simulink model "q_3d_crane_cal"  (Simulink 6.6)
settings: Solver=FixedStepDiscrete  StartTime=0.0  StopTime=inf  FixedStep=0.001  RelTol=1e-3
values from neighbouring files (symbols this model uses):
  calib_theta = 4.5*pi/180    (= 0.0785398163397)    [setup_3d_crane.m]
  calib_theta_dot = 1/1000    (= 0.001)    [setup_3d_crane.m]
  calib_x = 2/100    (= 0.02)    [setup_3d_crane.m]
  calib_x_dot = 2/1000    (= 0.002)    [setup_3d_crane.m]
  calib_z = 3/100    (= 0.03)    [setup_3d_crane.m]
  calib_z_dot = 5/1000    (= 0.005)    [setup_3d_crane.m]
  IMAX_AMP = 7    [setup_3d_crane.m]
  K_ENC_ALPHA = 2 * pi / (4 * 1024 )    (= 0.00153398078789)    [config_3d_crane.m]
  K_ENC_GAMMA = 2 * pi / (4 * 1024 )    (= 0.00153398078789)    [config_3d_crane.m]
  K_ENC_THETA = 2 * pi / (4 * 1024 ) / Kg_t    (= 1.53398078789e-05)    [config_3d_crane.m]
  K_ENC_X = - Pt / (4 * 1024 ) / Kg_j    [config_3d_crane.m]
  K_ENC_Z = - 2 * pi * r_y_reel / (4 * 1024 ) / Kg_y    [config_3d_crane.m]
  K_J = lqr(A_J,B_J,Q_J,R_J)    [setup_3d_crane.m]
  K_T = lqr(A_T,B_T,Q_T,R_T)    [setup_3d_crane.m]
  Ka = 0.5    [config_3d_crane.m]
  ki = w0^2*p0*(mp*r_y_reel^2+J_phi)/eff_g_y/Kg_y/eff_m_y/Kt_y/r_y_reel    [d_payload_piv_controller.m]
  kp = w0*(2*zeta*p0*J_phi+w0*mp*r_y_reel^2+w0*J_phi+2*zeta*p0*mp*r_y_reel^2)/eff_g_y/Kg_y/eff_m_y/Kt_y/r_y_reel    [d_payload_piv_controller.m]
  kv = (p0*J_phi+2*zeta*w0*mp*r_y_reel^2+2*zeta*w0*J_phi+p0*mp*r_y_reel^2)/eff_g_y/Kg_y/eff_m_y/Kt_y/r_y_reel    [d_payload_piv_controller.m]
  sp_home_payload = -0.7    [setup_3d_crane.m]
  sp_home_tower = 155    [setup_3d_crane.m]
  sp_home_trolley = 0.25    [setup_3d_crane.m]
  VMAX_DAC = 10    [setup_3d_crane.m]
  wf_gamma = 2 * pi * 2.0    (= 12.5663706144)    [setup_3d_crane.m]
  wf_theta = 2 * pi * 50    (= 314.159265359)    [setup_3d_crane.m]
  wf_x = 2 * pi * 50    (= 314.159265359)    [setup_3d_crane.m]
  wf_z = 2 * pi * 50    (= 314.159265359)    [setup_3d_crane.m]
undefined symbols (not defined in the file or in its folder): DiscIntNeverNeededParam, HIL, qc_get_step_size
libraries: quarc_library x21, simulink x14, simulink_extras x4
settings Model: Creator=MLevis  LastModifiedBy=MLevis  SimulationMode=external  ExtModeTrigDuration=25000
settings SolverCC: PositivePriorityOrder=on
settings RTWCC: SystemTargetFile=quarc_windows.tlc  TemplateMakefile=quarc_default_tmf  Description=QuaRC Win32 Target  ProcessScript=quarc_windows_make_rtw_hook
settings STFCustomTargetCC: TargetFcnLib=ansi_tfl_tmw.mat  TargetPreCompLibLocation=C:\DOCUME~1\ALLUSE~1\APPLIC~1\QUARC\lib\2007a\windows\release  GenFloatMathFcnCalls=ANSI_C  SystemTargetFile=quarc_windows.tlc
settings GRTTargetCC: TargetPreCompLibLocation=C:\DOCUME~1\ALLUSE~1\APPLIC~1\QUARC\lib\2007a\windows\release  MatFileLogging=off  ExtMode=on  ExtModeMexFile=quarc_comm

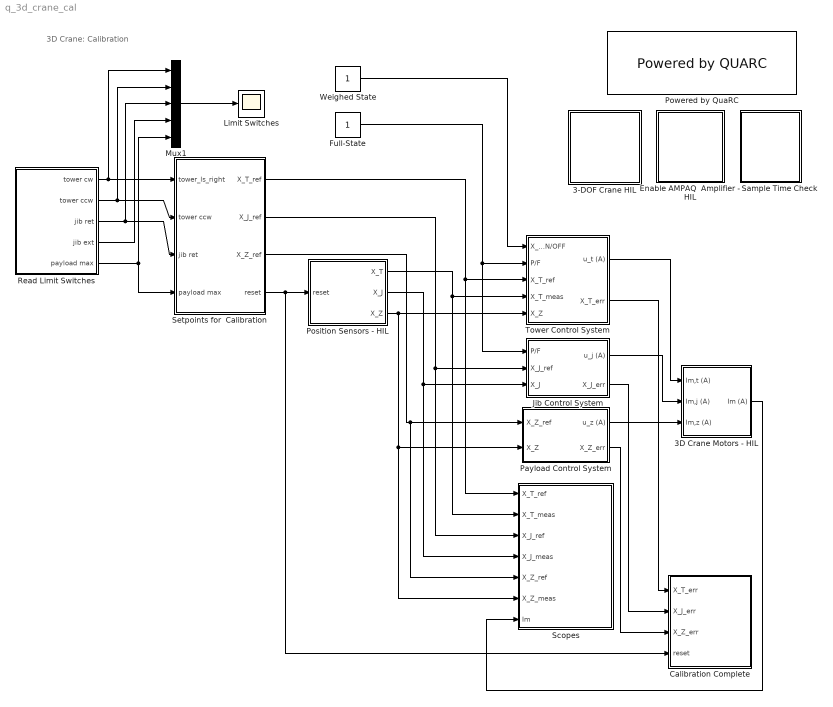
== system q_3d_crane_cal ==
  note: 3D Crane: Calibration
  3-DOF Crane HIL : Subsystem
  3D Crane Motors - HIL : Subsystem
  Calibration Complete : Subsystem
  Enable AMPAQ  Amplifier - HIL : Subsystem
  Full-State : Constant
  Jib Control System : Subsystem
  Limit Switches : Scope
      settings: TimeRange=25  YMin=-1  YMax=2  SaveName=ScopeData4
  Mux1 : Mux  Inputs=5
  Payload Control System : Subsystem
  Position Sensors - HIL : Subsystem
  Powered by QuaRC : quarc_library/Logos/Powered by QUARC  SystemSampleTime=-1
  Read Limit Switches : Subsystem
  Sample Time Check : Subsystem
  Scopes : Subsystem
  Setpoints for  Calibration : Subsystem
  Tower Control System : Subsystem
  Weighed State : Constant
  wires:
  Payload Control System/1(u_z (A)) -> 3D Crane Motors - HIL/3(Im,z (A))
  Tower Control System/1(u_t (A)) -> 3D Crane Motors - HIL/1(Im,t (A))
  Position Sensors - HIL/1(X_T) -> Scopes/2(X_T_meas), Tower Control System/4(X_T_meas)
  Position Sensors - HIL/3(X_Z) -> Scopes/6(X_Z_meas), Payload Control System/2(X_Z), Tower Control System/5(X_Z)
  Position Sensors - HIL/2(X_J) -> Scopes/4(X_J_meas), Jib Control System/3(X_J)
  Setpoints for  Calibration/2(X_J_ref) -> Scopes/3(X_J_ref), Jib Control System/2(X_J_ref)
  Setpoints for  Calibration/1(X_T_ref) -> Scopes/1(X_T_ref), Tower Control System/3(X_T_ref)
  Setpoints for  Calibration/3(X_Z_ref) -> Scopes/5(X_Z_ref), Payload Control System/1(X_Z_ref)
  Jib Control System/1(u_j (A)) -> 3D Crane Motors - HIL/2(Im,j (A))
  Weighed State/1 -> Tower Control System/1(X_W ON/OFF)
  3D Crane Motors - HIL/1(Im (A)) -> Scopes/7(Im)
  Full-State/1 -> Tower Control System/2(P/F), Jib Control System/1(P/F)
  Read Limit Switches/1(tower cw) -> Mux1/1, Setpoints for  Calibration/1(tower_ls_right)
  Read Limit Switches/3(jib ret) -> Mux1/3, Setpoints for  Calibration/3(jib ret)
  Read Limit Switches/5(payload max) -> Setpoints for  Calibration/4(payload max), Mux1/5
  Tower Control System/2(X_T_err) -> Calibration Complete/1(X_T_err)
  Jib Control System/2(X_J_err) -> Calibration Complete/2(X_J_err)
  Payload Control System/2(X_Z_err) -> Calibration Complete/3(X_Z_err)
  Setpoints for  Calibration/4(reset) -> Calibration Complete/4(reset), Position Sensors - HIL/1(reset)
  Read Limit Switches/4(jib ext) -> Mux1/4
  Read Limit Switches/2(tower ccw) -> Mux1/2, Setpoints for  Calibration/2(tower ccw)
  Mux1/1 -> Limit Switches/1

== system q_3d_crane_cal/3-DOF Crane HIL ==
  HIL Initialize : quarc_library/Data Acquisition/Generic/Configuration/HIL Initialize  object_name=HIL-1  board_type=q8  board_number=0  exclusive=off  active=on  hardware_clocks=[]  clock_modes=[]  initial_clock_frequencies=[]  set_clock_params_at_start=on  set_clock_params_at_switch_in=on  set_clock_frequencies_at_start=off  set_clock_frequencies_at_switch_in=off  analog_input_channels=[]  analog_input_maximums=[]  analog_input_minimums=[]  set_analog_input_params_at_start=on  set_analog_input_params_at_switch_in=on  analog_output_channels=[0:2]  analog_output_maximums=[10]  analog_output_minimums=[-10]  initial_analog_outputs=[0]  final_analog_outputs=[0]  watchdog_analog_outputs=0  set_analog_output_params_at_start=on  set_analog_output_params_at_switch_in=on  set_analog_outputs_at_start=on  set_analog_outputs_at_switch_in=off  set_analog_outputs_at_terminate=on  set_analog_outputs_at_switch_out=off  set_analog_outputs_on_watchdog=off  digital_input_channels=[8:11]  digital_output_channels=[0:2,4]  digital_output_configuration=[]  initial_digital_outputs=1  final_digital_outputs=1  watchdog_digital_outputs=0  set_digital_output_params_at_start=off  set_digital_output_params_at_switch_in=off  set_digital_outputs_at_start=on  set_digital_outputs_at_switch_in=off  set_digital_outputs_at_terminate=on  set_digital_outputs_at_switch_out=off  set_digital_outputs_on_watchdog=off  encoder_channels=[0:4]  quadrature=[4]  encoder_filter_frequency=[1/60e-9]  initial_encoder_counts=0  set_encoder_params_at_start=on  set_encoder_params_at_switch_in=on  set_encoder_counts_at_start=on  set_encoder_counts_at_switch_in=off  pwm_channels=[]  pwm_modes=[]  pwm_frequency=[]  pwm_configuration=[]  pwm_alignment=[]  pwm_polarity=[]  pwm_leading_deadband=[]  pwm_trailing_deadband=[]  initial_pwm_outputs=0  final_pwm_outputs=0  watchdog_pwm_outputs=0  set_pwm_params_at_start=on  set_pwm_params_at_switch_in=on  set_pwm_outputs_at_start=on  set_pwm_outputs_at_switch_in=off  set_pwm_outputs_at_terminate=on  set_pwm_outputs_at_switch_out=off  set_pwm_outputs_on_watchdog=off  other_output_channels=[]  initial_other_outputs=0  final_other_outputs=0  watchdog_other_outputs=0  set_other_outputs_at_start=on  set_other_outputs_at_switch_in=off  set_other_outputs_at_terminate=on  set_other_outputs_at_switch_out=off  set_other_outputs_on_watchdog=off
      settings: AttributesFormatString=%<object_name>
  HIL Read Timebase : quarc_library/Data Acquisition/Generic/Timebases/HIL Read Timebase  Tag=unassigned  object_name=HIL-1  clock=0  analog_channels=[0:2]  encoder_channels=[0:4]  digital_channels=[8:12]  other_channels=[]  samples_in_buffer=max(ceil(1/qc_get_step_size), 1)  active=on  vector_output=on  data_type_mode=Inherit via back propagation  encoder_data_type=double  digital_data_type=boolean
  HIL Write : quarc_library/Data Acquisition/Generic/Immediate I//O/HIL Write  Tag=unassigned  object_name=HIL-1  analog_channels=[0:2]  pwm_channels=[]  digital_channels=[0:2,4]  other_channels=[]  sample_time=-1  active=off  vector_input=on
  Signal Specification : SignalSpecification  DataType=double
  tag scope: AI=global, DI=global, ENC_CNT=global
  wires:
  HIL Read Timebase/3 -> [DI]
  HIL Read Timebase/1 -> [AI]
  HIL Read Timebase/2 -> [ENC_CNT]
  [DO] -> HIL Write/2
  [AO] -> Signal Specification/1
  Signal Specification/1 -> HIL Write/1

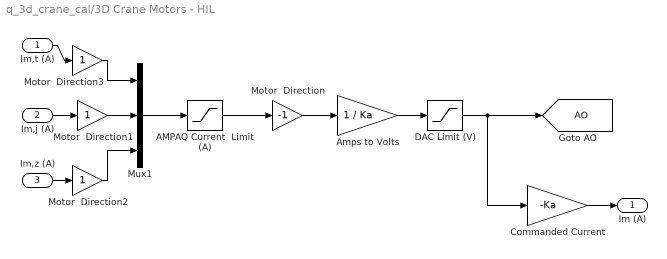
== system q_3d_crane_cal/3D Crane Motors - HIL ==
  Im,t (A) : Inport
  Im,j (A) : Inport  Port=2
  Im,z (A) : Inport  Port=3
  AMPAQ Current  Limit (A) : Saturate  UpperLimit=IMAX_AMP  LowerLimit=-IMAX_AMP
  Amps to Volts : Gain  Gain=1 / Ka  SaturateOnIntegerOverflow=on
  "Commanded Current " : Gain  Gain=-Ka  SaturateOnIntegerOverflow=on
  DAC Limit (V) : Saturate  UpperLimit=VMAX_DAC  LowerLimit=-VMAX_DAC
  Motor  Direction : Gain  Gain=-1
  Motor  Direction1 : Gain
  Motor  Direction2 : Gain
  Motor  Direction3 : Gain
  Mux1 : Mux  Inputs=3
  Im (A) : Outport
  tag scope: AO=global
  wires:
  Motor  Direction/1 -> Amps to Volts/1
  "Commanded Current "/1 -> Im (A)/1
  Mux1/1 -> AMPAQ Current  Limit (A)/1
  Im,z (A)/1 -> Motor  Direction2/1
  Im,j (A)/1 -> Motor  Direction1/1
  Im,t (A)/1 -> Motor  Direction3/1
  AMPAQ Current  Limit (A)/1 -> Motor  Direction/1
  DAC Limit (V)/1 -> "Commanded Current "/1, [AO]
  Amps to Volts/1 -> DAC Limit (V)/1
  Motor  Direction1/1 -> Mux1/2
  Motor  Direction2/1 -> Mux1/3
  Motor  Direction3/1 -> Mux1/1

== system q_3d_crane_cal/Calibration Complete ==
  note: Right Tower Limit Hit
  X_T_err : Inport
  X_J_err : Inport  Port=2
  X_Z_err : Inport  Port=3
  reset : Inport  Port=4
  All Encoders  Reset : Logic  Inputs=3  AllPortsSameDT=off  OutDataTypeMode=Boolean
  Cal Done : quarc_library/Sinks/Error Handling/Stop with Message  SystemSampleTime=-1  message_type=Fixed error message  message_icon=Information  message=Calibration complete.
  Demux : Demux  Outputs=3
  Enabled and Triggered Subsystem : Subsystem  TreatAsAtomicUnit=on
  Rate Transition : RateTransition
  System Calibrated : Logic  Inputs=3  AllPortsSameDT=off  OutDataTypeMode=Boolean
  Unit Delay : UnitDelay  SampleTime=4
  wires:
  System Calibrated/1 -> Cal Done/1
  Unit Delay/1 -> Enabled and Triggered Subsystem/Enable
  Enabled and Triggered Subsystem/3(payload_calib) -> System Calibrated/3
  Enabled and Triggered Subsystem/2(trolley_calib) -> System Calibrated/2
  Enabled and Triggered Subsystem/1(tower_calib) -> System Calibrated/1
  All Encoders  Reset/1 -> Rate Transition/1
  Demux/3 -> All Encoders  Reset/3
  Demux/2 -> All Encoders  Reset/2
  Demux/1 -> All Encoders  Reset/1
  X_Z_err/1 -> Enabled and Triggered Subsystem/3(X_Z_err)
  X_J_err/1 -> Enabled and Triggered Subsystem/2(X_J_err)
  X_T_err/1 -> Enabled and Triggered Subsystem/1(X_T_err)
  reset/1 -> Demux/1
  Rate Transition/1 -> Unit Delay/1

== system q_3d_crane_cal/Enable AMPAQ  Amplifier - HIL ==
  Enable Amp : Constant  Value=[0 0 0 1]
  tag scope: DO=global
  wires:
  Enable Amp/1 -> [DO]

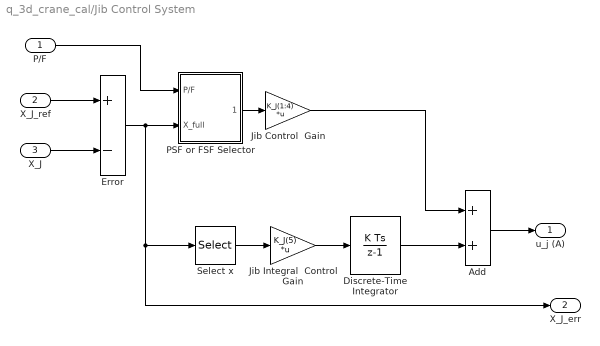
== system q_3d_crane_cal/Jib Control System ==
  P/F : Inport
  X_J_ref : Inport  Port=2
  X_J : Inport  Port=3
  Add : Sum  OutScaling=2^-10
  Discrete-Time Integrator : DiscreteIntegrator  SampleTime=qc_get_step_size  LimitOutput=on  UpperSaturationLimit=2  LowerSaturationLimit=-2  ICPrevOutput=DiscIntNeverNeededParam  ICPrevScaledInput=DiscIntNeverNeededParam
  Error : Sum  Inputs=+-  OutScaling=2^-10
  Jib Control  Gain : Gain  Gain=K_J(1:4)  Multiplication=Matrix(K*u)
  Jib Integral  Control Gain : Gain  Gain=K_J(5)  Multiplication=Matrix(K*u)
  PSF or FSF Selector : Subsystem
  Select x : Selector  IndexOptions=Index vector (dialog)  Indices=1  OutputSizes=1  InputPortWidth=4
  u_j (A) : Outport
  X_J_err : Outport  Port=2
  wires:
  PSF or FSF Selector/1(X_out) -> Jib Control  Gain/1
  P/F/1 -> PSF or FSF Selector/1(P/F)
  Add/1 -> u_j (A)/1
  Discrete-Time Integrator/1 -> Add/2
  Jib Control  Gain/1 -> Add/1
  Jib Integral  Control Gain/1 -> Discrete-Time Integrator/1
  Select x/1 -> Jib Integral  Control Gain/1
  X_J/1 -> Error/2
  X_J_ref/1 -> Error/1
  Error/1 -> PSF or FSF Selector/2(X_full), Select x/1, X_J_err/1

== system q_3d_crane_cal/Payload Control System ==
  X_Z_ref : Inport
  X_Z : Inport  Port=2
  Add : Sum  Inputs=+++  OutScaling=2^-10
  Demux : Demux  Outputs=2
  Discrete-Time Integrator : DiscreteIntegrator  SampleTime=qc_get_step_size  ICPrevOutput=DiscIntNeverNeededParam  ICPrevScaledInput=DiscIntNeverNeededParam
  Payload Integral  Gain : Gain  Gain=ki
  Payload Proportional  Gain : Gain  Gain=kp
  Payload Velocity  Gain : Gain  Gain=kv
  Subtract : Sum  Inputs=+-  OutScaling=2^-10
  u_z (A) : Outport
  X_Z_err : Outport  Port=2
  wires:
  X_Z/1 -> Subtract/2
  X_Z_ref/1 -> Subtract/1
  Payload Integral  Gain/1 -> Discrete-Time Integrator/1
  Add/1 -> u_z (A)/1
  Payload Proportional  Gain/1 -> Add/1
  Discrete-Time Integrator/1 -> Add/2
  Subtract/1 -> Demux/1, X_Z_err/1
  Demux/1 -> Payload Proportional  Gain/1, Payload Integral  Gain/1
  Demux/2 -> Payload Velocity  Gain/1
  Payload Velocity  Gain/1 -> Add/3

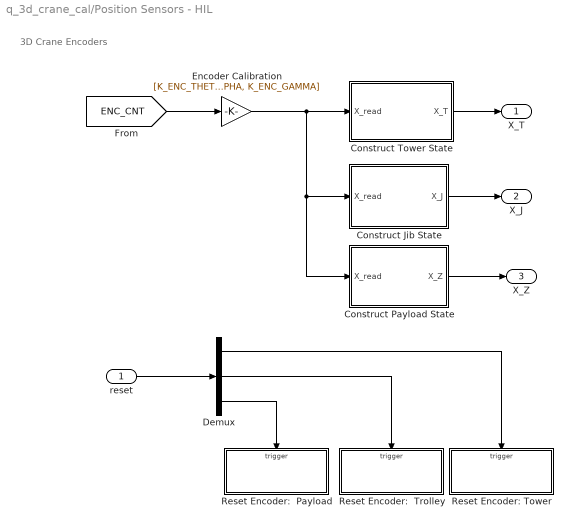
== system q_3d_crane_cal/Position Sensors - HIL ==
  note: 3D Crane Encoders
  reset : Inport
  Construct Jib State : Subsystem
  Construct Payload State : Subsystem
  Construct Tower State : Subsystem
  Demux : Demux  Outputs=3
  Encoder Calibration : Gain  Gain=[K_ENC_THETA, K_ENC_X, K_ENC_Z, K_ENC_ALPHA, K_ENC_GAMMA]
  Reset Encoder: Tower : Subsystem  TreatAsAtomicUnit=on
  Reset Encoder:  Payload : Subsystem  TreatAsAtomicUnit=on
  Reset Encoder:  Trolley : Subsystem  TreatAsAtomicUnit=on
  X_T : Outport
  X_J : Outport  Port=2
  X_Z : Outport  Port=3
  wires:
  [ENC_CNT] -> Encoder Calibration/1
  Encoder Calibration/1 -> Construct Tower State/1(X_read), Construct Jib State/1(X_read), Construct Payload State/1(X_read)
  Construct Tower State/1(X_T) -> X_T/1
  Construct Jib State/1(X_J) -> X_J/1
  Construct Payload State/1(X_Z) -> X_Z/1
  Demux/1 -> Reset Encoder: Tower/Trigger
  Demux/2 -> Reset Encoder:  Trolley/Trigger
  Demux/3 -> Reset Encoder:  Payload/Trigger
  reset/1 -> Demux/1

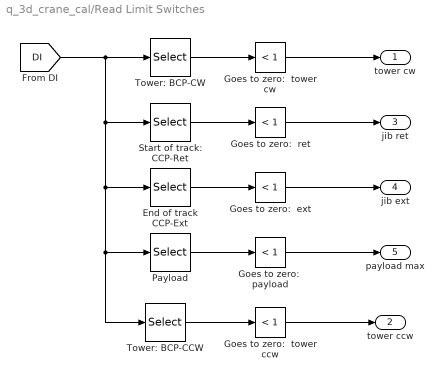
== system q_3d_crane_cal/Read Limit Switches ==
  End of track CCP-Ext : Selector  IndexOptions=Index vector (dialog)  Indices=3  OutputSizes=1  InputPortWidth=5
  Goes to zero:  ext : simulink/Logic and Bit Operations/Compare To Constant  SystemSampleTime=-1  relop=<  const=1  LogicOutDataTypeMode=boolean  ZeroCross=off
  Goes to zero:  payload : simulink/Logic and Bit Operations/Compare To Constant  SystemSampleTime=-1  relop=<  const=1  LogicOutDataTypeMode=boolean  ZeroCross=off
  Goes to zero:  ret : simulink/Logic and Bit Operations/Compare To Constant  SystemSampleTime=-1  relop=<  const=1  LogicOutDataTypeMode=boolean  ZeroCross=off
  Goes to zero:  tower ccw : simulink/Logic and Bit Operations/Compare To Constant  SystemSampleTime=-1  relop=<  const=1  LogicOutDataTypeMode=boolean  ZeroCross=off
  Goes to zero:  tower cw : simulink/Logic and Bit Operations/Compare To Constant  SystemSampleTime=-1  relop=<  const=1  LogicOutDataTypeMode=boolean  ZeroCross=off
  Payload : Selector  IndexOptions=Index vector (dialog)  Indices=4  OutputSizes=1  InputPortWidth=5
  Start of track: CCP-Ret : Selector  IndexOptions=Index vector (dialog)  Indices=2  OutputSizes=1  InputPortWidth=5
  Tower: BCP-CCW : Selector  IndexOptions=Index vector (dialog)  Indices=5  OutputSizes=1  InputPortWidth=5
  Tower: BCP-CW : Selector  IndexOptions=Index vector (dialog)  Indices=1  OutputSizes=1  InputPortWidth=5
  tower cw : Outport
  tower ccw : Outport  Port=2
  jib ret : Outport  Port=3
  jib ext : Outport  Port=4
  payload max : Outport  Port=5
  wires:
  Goes to zero:  tower ccw/1 -> tower ccw/1
  Tower: BCP-CCW/1 -> Goes to zero:  tower ccw/1
  End of track CCP-Ext/1 -> Goes to zero:  ext/1
  Start of track: CCP-Ret/1 -> Goes to zero:  ret/1
  Goes to zero:  ext/1 -> jib ext/1
  Goes to zero:  ret/1 -> jib ret/1
  Tower: BCP-CW/1 -> Goes to zero:  tower cw/1
  Goes to zero:  tower cw/1 -> tower cw/1
  Goes to zero:  payload/1 -> payload max/1
  Payload/1 -> Goes to zero:  payload/1
  [DI] -> Tower: BCP-CW/1, Start of track: CCP-Ret/1, Tower: BCP-CCW/1, Payload/1, End of track CCP-Ext/1

== system q_3d_crane_cal/Sample Time Check ==
  Larger than  2x sample time? : simulink/Logic and Bit Operations/Compare To Constant  SystemSampleTime=-1  relop=>  const=2*qc_get_step_size  LogicOutDataTypeMode=uint8  ZeroCross=off
  Max Missed Samples : simulink/Logic and Bit Operations/Compare To Constant  SystemSampleTime=-1  relop=>  const=5  LogicOutDataTypeMode=uint8  ZeroCross=off
  Memory : Memory  Orientation=left
  Sample Time : quarc_library/Sources/Time/Sample Time  Priority=-99  sample_time=qc_get_step_size
  Samples Missed : Display
  Stop with Message : quarc_library/Sinks/Error Handling/Stop with Message  SystemSampleTime=-1  message_type=Fixed error message  message_icon=Error  message=Maximum number of missed samples reached. Please reduce your CPU load.
  Sum : Sum  Inputs=|++
  wires:
  Sample Time/1 -> Larger than  2x sample time?/1
  Larger than  2x sample time?/1 -> Sum/1
  Sum/1 -> Samples Missed/1, Max Missed Samples/1, Memory/1
  Memory/1 -> Sum/2
  Max Missed Samples/1 -> Stop with Message/1

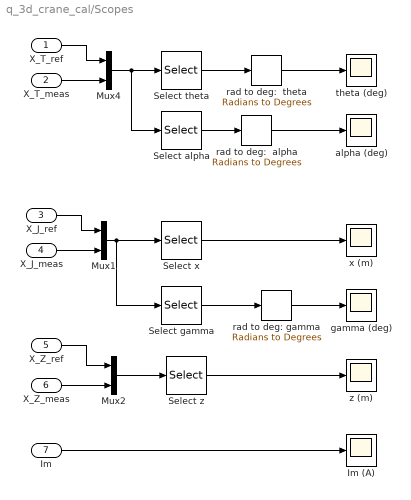
== system q_3d_crane_cal/Scopes ==
  X_T_ref : Inport
  X_T_meas : Inport  Port=2
  X_J_ref : Inport  Port=3
  X_J_meas : Inport  Port=4
  X_Z_ref : Inport  Port=5
  X_Z_meas : Inport  Port=6
  Im : Inport  Port=7
  Im (A) : Scope
      settings: TimeRange=25  SaveName=ScopeData3
  Mux1 : Mux  Inputs=2
  Mux2 : Mux  Inputs=2
  Mux4 : Mux  Inputs=2
  Select alpha : Selector  IndexOptions=Index vector (dialog)  Indices=[2 6]  OutputSizes=1  InputPortWidth=8
  Select gamma : Selector  IndexOptions=Index vector (dialog)  Indices=[2 6]  OutputSizes=1  InputPortWidth=8
  Select theta : Selector  IndexOptions=Index vector (dialog)  Indices=[1 5]  OutputSizes=1  InputPortWidth=8
  Select x : Selector  IndexOptions=Index vector (dialog)  Indices=[1 5]  OutputSizes=1  InputPortWidth=8
  Select z : Selector  IndexOptions=Index vector (dialog)  Indices=[1 3]  OutputSizes=1  InputPortWidth=4
  alpha (deg) : Scope
      settings: TimeRange=25
  gamma (deg) : Scope
      settings: TimeRange=25  SaveName=ScopeData9
  rad to deg:  theta : simulink_extras/Transformations/Radians to Degrees  SystemSampleTime=-1
  rad to deg: gamma : simulink_extras/Transformations/Radians to Degrees  SystemSampleTime=-1
  rad to deg:  alpha : simulink_extras/Transformations/Radians to Degrees  SystemSampleTime=-1
  theta (deg) : Scope
      settings: TimeRange=25  YMin=-25  YMax=175  SaveName=ScopeData8
  x (m) : Scope
      settings: TimeRange=25  YMin=-1  YMax=1
  z (m) : Scope
      settings: TimeRange=25  YMin=-0.1  YMax=0.9  SaveName=ScopeData2
  wires:
  Im/1 -> Im (A)/1
  rad to deg:  theta/1 -> theta (deg)/1
  rad to deg: gamma/1 -> gamma (deg)/1
  rad to deg:  alpha/1 -> alpha (deg)/1
  Select theta/1 -> rad to deg:  theta/1
  X_T_ref/1 -> Mux4/1
  Mux4/1 -> Select theta/1, Select alpha/1
  Select x/1 -> x (m)/1
  Mux2/1 -> Select z/1
  Select alpha/1 -> rad to deg:  alpha/1
  Select gamma/1 -> rad to deg: gamma/1
  X_J_ref/1 -> Mux1/1
  X_J_meas/1 -> Mux1/2
  Mux1/1 -> Select x/1, Select gamma/1
  X_Z_ref/1 -> Mux2/1
  X_Z_meas/1 -> Mux2/2
  Select z/1 -> z (m)/1
  X_T_meas/1 -> Mux4/2

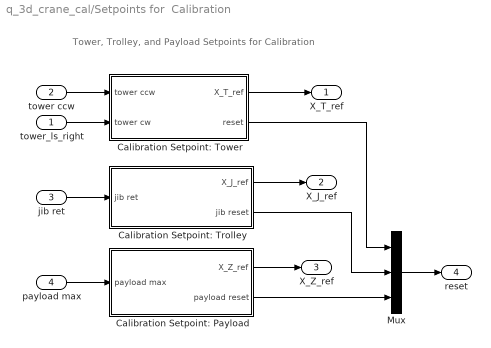
== system q_3d_crane_cal/Setpoints for  Calibration ==
  note: Tower, Trolley, and Payload Setpoints for Calibration
  tower_ls_right : Inport
  tower ccw : Inport  Port=2
  jib ret : Inport  Port=3
  payload max : Inport  Port=4
  Calibration Setpoint: Payload : Subsystem
  Calibration Setpoint: Tower : Subsystem
  Calibration Setpoint: Trolley : Subsystem
  Mux : Mux  Inputs=3
  X_T_ref : Outport
  X_J_ref : Outport  Port=2
  X_Z_ref : Outport  Port=3
  reset : Outport  Port=4
  wires:
  tower_ls_right/1 -> Calibration Setpoint: Tower/2(tower cw)
  payload max/1 -> Calibration Setpoint: Payload/1(payload max)
  jib ret/1 -> Calibration Setpoint: Trolley/1(jib ret)
  tower ccw/1 -> Calibration Setpoint: Tower/1(tower ccw)
  Mux/1 -> reset/1
  Calibration Setpoint: Payload/2(payload reset) -> Mux/3
  Calibration Setpoint: Payload/1(X_Z_ref) -> X_Z_ref/1
  Calibration Setpoint: Trolley/2(jib reset) -> Mux/2
  Calibration Setpoint: Trolley/1(X_J_ref) -> X_J_ref/1
  Calibration Setpoint: Tower/2(reset) -> Mux/1
  Calibration Setpoint: Tower/1(X_T_ref) -> X_T_ref/1

== system q_3d_crane_cal/Tower Control System ==
  X_W ON/OFF : Inport
  P/F : Inport  Port=2
  X_T_ref : Inport  Port=3
  X_T_meas : Inport  Port=4
  X_Z : Inport  Port=5
  PSF or FSF Selector : Subsystem
  Tower Control  Gain : Gain  Gain=K_T  Multiplication=Matrix(K*u)
  Tower Error : Sum  Inputs=+-  OutScaling=2^-10
  Weighed State : Subsystem
  u_t (A) : Outport
  X_T_err : Outport  Port=2
  wires:
  Tower Control  Gain/1 -> u_t (A)/1
  X_T_ref/1 -> Tower Error/1
  X_T_meas/1 -> Tower Error/2
  P/F/1 -> PSF or FSF Selector/1(P/F)
  Tower Error/1 -> PSF or FSF Selector/2(X_full), X_T_err/1
  X_Z/1 -> Weighed State/1(X_Z)
  X_W ON/OFF/1 -> Weighed State/2(X_W ON/OFF)
  PSF or FSF Selector/1(X_out) -> Weighed State/3(X_in)
  Weighed State/1(X_w) -> Tower Control  Gain/1

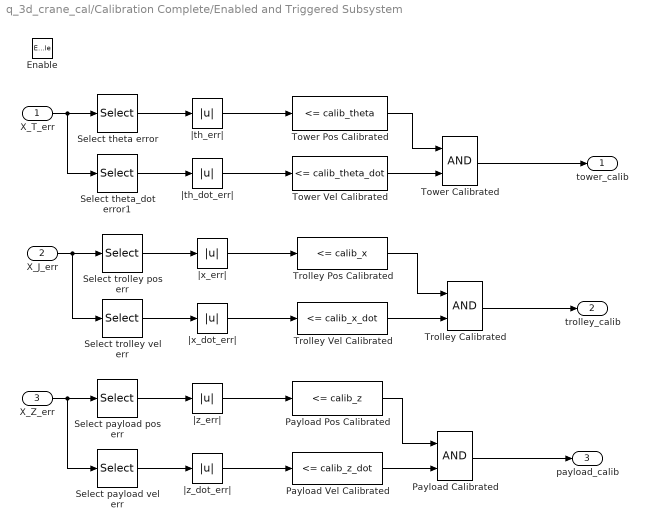
== system q_3d_crane_cal/Calibration Complete/Enabled and Triggered Subsystem ==
  X_T_err : Inport
  X_J_err : Inport  Port=2
  X_Z_err : Inport  Port=3
  Enable : EnablePort
  Payload Calibrated : Logic  AllPortsSameDT=off  OutDataTypeMode=Boolean
  Payload Pos Calibrated : simulink/Logic and Bit Operations/Compare To Constant  SystemSampleTime=-1  relop=<=  const=calib_z  LogicOutDataTypeMode=uint8  ZeroCross=off
  Payload Vel Calibrated : simulink/Logic and Bit Operations/Compare To Constant  SystemSampleTime=-1  relop=<=  const=calib_z_dot  LogicOutDataTypeMode=uint8  ZeroCross=off
  Select payload pos err : Selector  IndexOptions=Index vector (dialog)  Indices=1  OutputSizes=1  InputPortWidth=2
  Select payload vel err : Selector  IndexOptions=Index vector (dialog)  Indices=2  OutputSizes=1  InputPortWidth=2
  Select theta error : Selector  IndexOptions=Index vector (dialog)  Indices=1  OutputSizes=1  InputPortWidth=4
  Select theta_dot error1 : Selector  IndexOptions=Index vector (dialog)  Indices=3  OutputSizes=1  InputPortWidth=4
  Select trolley pos err : Selector  IndexOptions=Index vector (dialog)  Indices=1  OutputSizes=1  InputPortWidth=4
  Select trolley vel err : Selector  IndexOptions=Index vector (dialog)  Indices=3  OutputSizes=1  InputPortWidth=4
  Tower Calibrated : Logic  AllPortsSameDT=off  OutDataTypeMode=Boolean
  Tower Pos Calibrated : simulink/Logic and Bit Operations/Compare To Constant  SystemSampleTime=-1  relop=<=  const=calib_theta  LogicOutDataTypeMode=uint8  ZeroCross=off
  Tower Vel Calibrated : simulink/Logic and Bit Operations/Compare To Constant  SystemSampleTime=-1  relop=<=  const=calib_theta_dot  LogicOutDataTypeMode=uint8  ZeroCross=off
  Trolley Calibrated : Logic  AllPortsSameDT=off  OutDataTypeMode=Boolean
  Trolley Pos Calibrated : simulink/Logic and Bit Operations/Compare To Constant  SystemSampleTime=-1  relop=<=  const=calib_x  LogicOutDataTypeMode=uint8  ZeroCross=off
  Trolley Vel Calibrated : simulink/Logic and Bit Operations/Compare To Constant  SystemSampleTime=-1  relop=<=  const=calib_x_dot  LogicOutDataTypeMode=uint8  ZeroCross=off
  |th_dot_err| : Abs
  |th_err| : Abs
  |x_dot_err| : Abs
  |x_err| : Abs
  |z_dot_err| : Abs
  |z_err| : Abs
  tower_calib : Outport
  trolley_calib : Outport  Port=2
  payload_calib : Outport  Port=3
  wires:
  Payload Calibrated/1 -> payload_calib/1
  Payload Vel Calibrated/1 -> Payload Calibrated/2
  Payload Pos Calibrated/1 -> Payload Calibrated/1
  Trolley Calibrated/1 -> trolley_calib/1
  Trolley Vel Calibrated/1 -> Trolley Calibrated/2
  Trolley Pos Calibrated/1 -> Trolley Calibrated/1
  Tower Calibrated/1 -> tower_calib/1
  Tower Vel Calibrated/1 -> Tower Calibrated/2
  Tower Pos Calibrated/1 -> Tower Calibrated/1
  |z_dot_err|/1 -> Payload Vel Calibrated/1
  Select payload vel err/1 -> |z_dot_err|/1
  |x_dot_err|/1 -> Trolley Vel Calibrated/1
  |th_dot_err|/1 -> Tower Vel Calibrated/1
  Select trolley vel err/1 -> |x_dot_err|/1
  Select theta_dot error1/1 -> |th_dot_err|/1
  X_Z_err/1 -> Select payload vel err/1, Select payload pos err/1
  X_J_err/1 -> Select trolley vel err/1, Select trolley pos err/1
  |x_err|/1 -> Trolley Pos Calibrated/1
  |z_err|/1 -> Payload Pos Calibrated/1
  Select payload pos err/1 -> |z_err|/1
  Select trolley pos err/1 -> |x_err|/1
  X_T_err/1 -> Select theta_dot error1/1, Select theta error/1
  |th_err|/1 -> Tower Pos Calibrated/1
  Select theta error/1 -> |th_err|/1

== system q_3d_crane_cal/Jib Control System/PSF or FSF Selector ==
  note: Partial-state or Full-state Feedback
  note: 0 = partial and 1 = full,
  note: state
  note: control input
  P/F : Inport
  X_full : Inport  Port=2
  Constant: FS : Constant  Value=[1 1 1 1]
  Constant: PS : Constant  Value=[1 0 1 0]
  Full-state : Product  RndMeth=Zero
  Multiport Switch : MultiPortSwitch  Inputs=2  zeroidx=on
  Partial-state : Product  RndMeth=Zero
  X_out : Outport
  wires:
  Constant: FS/1 -> Full-state/2
  Constant: PS/1 -> Partial-state/1
  Partial-state/1 -> Multiport Switch/2
  Full-state/1 -> Multiport Switch/3
  Multiport Switch/1 -> X_out/1
  P/F/1 -> Multiport Switch/1
  X_full/1 -> Partial-state/2, Full-state/1

== system q_3d_crane_cal/Position Sensors - HIL/Construct Jib State ==
  note: Jib State
  X_read : Inport
  Demux2 : Demux  Outputs=2
  High-Pass Filter: gamma : quarc_library/Discrete/Discretized Transfer Function  SystemSampleTime=-1  num=[wf_gamma 0]  den=[1 wf_gamma]  method=tustin  Ts=qc_get_step_size
  High-Pass Filter: x : quarc_library/Discrete/Discretized Transfer Function  SystemSampleTime=-1  num=[wf_x 0]  den=[1 wf_x]  method=tustin  Ts=qc_get_step_size
  Low-Pass Filter: gamma : quarc_library/Discrete/Discretized Transfer Function  SystemSampleTime=-1  num=[wf_gamma]  den=[1 wf_gamma]  method=tustin  Ts=qc_get_step_size
  Low-Pass Filter: x : quarc_library/Discrete/Discretized Transfer Function  SystemSampleTime=-1  num=[wf_x]  den=[1 wf_x]  method=tustin  Ts=qc_get_step_size
  Mux1 : Mux
  Select x and gamma : Selector  IndexOptions=Index vector (dialog)  Indices=[2, 5]  OutputSizes=1  InputPortWidth=5
  X_J : Outport
  wires:
  Mux1/1 -> X_J/1
  Select x and gamma/1 -> Demux2/1
  X_read/1 -> Select x and gamma/1
  Demux2/1 -> Low-Pass Filter: x/1, High-Pass Filter: x/1
  Demux2/2 -> Low-Pass Filter: gamma/1, High-Pass Filter: gamma/1
  Low-Pass Filter: x/1 -> Mux1/1
  Low-Pass Filter: gamma/1 -> Mux1/2
  High-Pass Filter: x/1 -> Mux1/3
  High-Pass Filter: gamma/1 -> Mux1/4

== system q_3d_crane_cal/Position Sensors - HIL/Construct Payload State ==
  note: Payload State
  X_read : Inport
  High-Pass Filter: z : quarc_library/Discrete/Discretized Transfer Function  SystemSampleTime=-1  num=[wf_z 0]  den=[1 wf_z]  method=tustin  Ts=qc_get_step_size
  Mux2 : Mux  Inputs=2
  Select z : Selector  IndexOptions=Index vector (dialog)  Indices=3  OutputSizes=1  InputPortWidth=5
  X_Z : Outport
  wires:
  Select z/1 -> Mux2/1, High-Pass Filter: z/1
  Mux2/1 -> X_Z/1
  X_read/1 -> Select z/1
  High-Pass Filter: z/1 -> Mux2/2

== system q_3d_crane_cal/Position Sensors - HIL/Construct Tower State ==
  note: Tower State
  X_read : Inport
  Demux1 : Demux  Outputs=2
  High-Pass Filter: alpha : quarc_library/Discrete/Discretized Transfer Function  SystemSampleTime=-1  num=[wf_gamma 0]  den=[1 wf_gamma]  method=tustin  Ts=qc_get_step_size
  High-Pass Filter: theta : quarc_library/Discrete/Discretized Transfer Function  SystemSampleTime=-1  num=[wf_theta 0]  den=[1 wf_theta]  method=tustin  Ts=qc_get_step_size
  Mux : Mux
  Select Theta and Alpha : Selector  IndexOptions=Index vector (dialog)  Indices=[1, 4]  OutputSizes=1  InputPortWidth=5
  X_T : Outport
  wires:
  Mux/1 -> X_T/1
  Select Theta and Alpha/1 -> Demux1/1
  X_read/1 -> Select Theta and Alpha/1
  Demux1/1 -> Mux/1, High-Pass Filter: theta/1
  Demux1/2 -> Mux/2, High-Pass Filter: alpha/1
  High-Pass Filter: theta/1 -> Mux/3
  High-Pass Filter: alpha/1 -> Mux/4

== system q_3d_crane_cal/Position Sensors - HIL/Reset Encoder: Tower ==
  Trigger : TriggerPort
  HIL Set Encoder Counts : quarc_library/Data Acquisition/Generic/Configuration/HIL Set Encoder Counts  object_name=HIL-1  channels=0  source=internal  counts=0  sample_time=-1  active=on  vector_input=off
      settings: AttributesFormatString=(%<object_name>)

== system q_3d_crane_cal/Position Sensors - HIL/Reset Encoder:  Payload ==
  Trigger : TriggerPort
  HIL Set Encoder Counts : quarc_library/Data Acquisition/Generic/Configuration/HIL Set Encoder Counts  object_name=HIL-1  channels=2  source=internal  counts=0  sample_time=-1  active=on  vector_input=off
      settings: AttributesFormatString=(%<object_name>)

== system q_3d_crane_cal/Position Sensors - HIL/Reset Encoder:  Trolley ==
  Trigger : TriggerPort
  HIL Set Encoder Counts : quarc_library/Data Acquisition/Generic/Configuration/HIL Set Encoder Counts  object_name=HIL-1  channels=1  source=internal  counts=0  sample_time=-1  active=on  vector_input=off
      settings: AttributesFormatString=(%<object_name>)

== system q_3d_crane_cal/Setpoints for  Calibration/Calibration Setpoint: Payload ==
  note: Spool up, reseet encoder, and bring down to 0.70 meters.
  note: X_Z = [z_ref,0,0,0]^T
  payload max : Inport
  Initial Setpoint:  Trolley : Constant  Value=0
  Multiport Switch : MultiPortSwitch  Inputs=2  zeroidx=on
  Mux2 : Mux  Inputs=3
  Payload Setpoint  Vector : Gain  Gain=[1, 0]
  Setpoint Calibration: Payload : Subsystem
  Terminator : Terminator
  Triggered Sigmoid : quarc_library/Sources/Sigmoids/Triggered Sigmoid  SystemSampleTime=-1  params_source=Internal (dialog parameters)  max_velocity=0.25  max_acceleration=0.25  hold_off=0.5  output_sample_time=qc_get_step_size  trigger=rising
  X_Z_ref : Outport
  payload reset : Outport  Port=2
  wires:
  Setpoint Calibration: Payload/1(reset) -> Triggered Sigmoid/1, payload reset/1, Multiport Switch/1
  payload max/1 -> Setpoint Calibration: Payload/1(ls payload)
  Initial Setpoint:  Trolley/1 -> Triggered Sigmoid/2, Triggered Sigmoid/3
  Triggered Sigmoid/4 -> Mux2/3
  Triggered Sigmoid/3 -> Mux2/2
  Triggered Sigmoid/2 -> Mux2/1
  Multiport Switch/1 -> Payload Setpoint  Vector/1
  Setpoint Calibration: Payload/2(xd) -> Multiport Switch/2, Triggered Sigmoid/4
  Payload Setpoint  Vector/1 -> X_Z_ref/1
  Mux2/1 -> Terminator/1
  Triggered Sigmoid/1 -> Multiport Switch/3

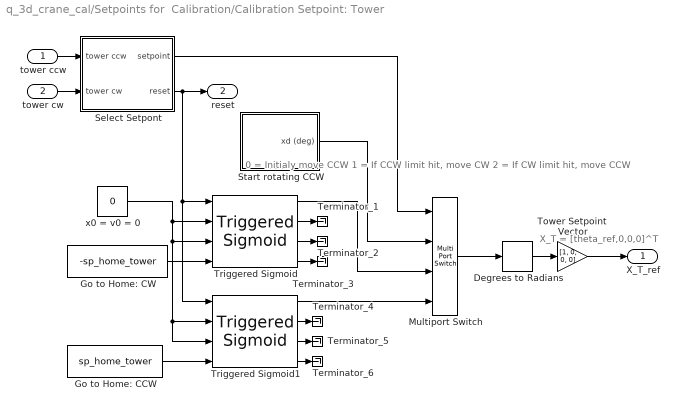
== system q_3d_crane_cal/Setpoints for  Calibration/Calibration Setpoint: Tower ==
  note: X_T = [theta_ref,0,0,0]^T
  note: 0 = Initialy move CCW
      | 1 = If CCW limit hit, move CW
      | 2 = If CW limit hit, move CCW
  tower ccw : Inport
  tower cw : Inport  Port=2
  Degrees to Radians : simulink_extras/Transformations/Degrees to Radians  SystemSampleTime=-1
  Go to Home: CCW : Constant  Value=sp_home_tower
  Go to Home: CW : Constant  Value=-sp_home_tower
  Multiport Switch : MultiPortSwitch  Inputs=3  zeroidx=on
  Select Setpont : Subsystem
  Start rotating CCW : Subsystem
  Terminator_{1..6} (6 alike) : Terminator
  Tower Setpoint  Vector : Gain  Gain=[1, 0, 0, 0]
  Triggered Sigmoid : quarc_library/Sources/Sigmoids/Triggered Sigmoid  SystemSampleTime=-1  params_source=Internal (dialog parameters)  max_velocity=75  max_acceleration=45  hold_off=0.5  output_sample_time=qc_get_step_size  trigger=rising
  Triggered Sigmoid1 : quarc_library/Sources/Sigmoids/Triggered Sigmoid  SystemSampleTime=-1  params_source=Internal (dialog parameters)  max_velocity=75  max_acceleration=45  hold_off=0.5  output_sample_time=qc_get_step_size  trigger=rising
  x0 = v0 = 0 : Constant  Value=0
  X_T_ref : Outport
  reset : Outport  Port=2  InitialOutput=0
  wires:
  Degrees to Radians/1 -> Tower Setpoint  Vector/1
  Tower Setpoint  Vector/1 -> X_T_ref/1
  Select Setpont/1(setpoint) -> Multiport Switch/1
  Start rotating CCW/1(xd (deg)) -> Multiport Switch/2
  Triggered Sigmoid/2 -> Terminator_1/1
  Triggered Sigmoid/3 -> Terminator_2/1
  Triggered Sigmoid/4 -> Terminator_3/1
  Go to Home: CW/1 -> Triggered Sigmoid/4
  Triggered Sigmoid1/2 -> Terminator_4/1
  Triggered Sigmoid1/3 -> Terminator_5/1
  Triggered Sigmoid1/4 -> Terminator_6/1
  Go to Home: CCW/1 -> Triggered Sigmoid1/4
  Triggered Sigmoid/1 -> Multiport Switch/3
  Triggered Sigmoid1/1 -> Multiport Switch/4
  Multiport Switch/1 -> Degrees to Radians/1
  tower ccw/1 -> Select Setpont/1(tower ccw)
  tower cw/1 -> Select Setpont/2(tower cw)
  Select Setpont/2(reset) -> reset/1, Triggered Sigmoid/1, Triggered Sigmoid1/1
  x0 = v0 = 0/1 -> Triggered Sigmoid/3, Triggered Sigmoid1/3, Triggered Sigmoid1/2, Triggered Sigmoid/2

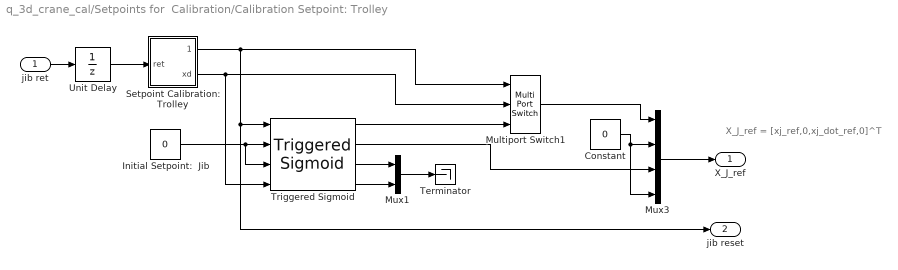
== system q_3d_crane_cal/Setpoints for  Calibration/Calibration Setpoint: Trolley ==
  note: X_J_ref = [xj_ref,0,xj_dot_ref,0]^T
  jib ret : Inport
  Constant : Constant  Value=0
  Initial Setpoint:  Jib : Constant  Value=0
  Multiport Switch1 : MultiPortSwitch  Inputs=2  zeroidx=on
  Mux1 : Mux  Inputs=2
  Mux3 : Mux
  Setpoint Calibration: Trolley : Subsystem
  Terminator : Terminator
  Triggered Sigmoid : quarc_library/Sources/Sigmoids/Triggered Sigmoid  SystemSampleTime=-1  params_source=Internal (dialog parameters)  max_velocity=0.75  max_acceleration=1.5  hold_off=0.5  output_sample_time=qc_get_step_size  trigger=rising
  Unit Delay : UnitDelay  SampleTime=qc_get_step_size
  X_J_ref : Outport
  jib reset : Outport  Port=2
  wires:
  Unit Delay/1 -> Setpoint Calibration: Trolley/1(ret)
  jib ret/1 -> Unit Delay/1
  Triggered Sigmoid/2 -> Mux3/3
  Constant/1 -> Mux3/4, Mux3/2
  Triggered Sigmoid/1 -> Multiport Switch1/3
  Multiport Switch1/1 -> Mux3/1
  Initial Setpoint:  Jib/1 -> Triggered Sigmoid/2, Triggered Sigmoid/3
  Setpoint Calibration: Trolley/2(xd) -> Multiport Switch1/2, Triggered Sigmoid/4
  Setpoint Calibration: Trolley/1(reset) -> jib reset/1, Triggered Sigmoid/1, Multiport Switch1/1
  Triggered Sigmoid/4 -> Mux1/2
  Triggered Sigmoid/3 -> Mux1/1
  Mux3/1 -> X_J_ref/1
  Mux1/1 -> Terminator/1

== system q_3d_crane_cal/Tower Control System/PSF or FSF Selector ==
  note: control input
  note: state
  note: 0 = partial and 1 = full,
  note: Partial-state or Full-state Feedback
  P/F : Inport
  X_full : Inport  Port=2
  Constant: FS : Constant  Value=[1 1 1 1]
  Constant: PS : Constant  Value=[1 0 1 0]
  Full-state : Product  RndMeth=Zero
  Multiport Switch : MultiPortSwitch  Inputs=2  zeroidx=on
  Partial-state : Product  RndMeth=Zero
  X_out : Outport
  wires:
  X_full/1 -> Full-state/1, Partial-state/2
  P/F/1 -> Multiport Switch/1
  Multiport Switch/1 -> X_out/1
  Full-state/1 -> Multiport Switch/3
  Partial-state/1 -> Multiport Switch/2
  Constant: PS/1 -> Partial-state/1
  Constant: FS/1 -> Full-state/2

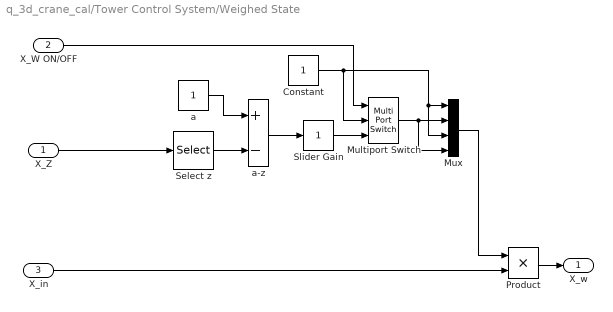
== system q_3d_crane_cal/Tower Control System/Weighed State ==
  X_Z : Inport
  X_W ON/OFF : Inport  Port=2
  X_in : Inport  Port=3
  Constant : Constant
  Multiport Switch : MultiPortSwitch  Inputs=2  zeroidx=on
  Mux : Mux
  Product : Product  RndMeth=Zero
  Select z : Selector  IndexOptions=Index vector (dialog)  Indices=1  OutputSizes=1  InputPortWidth=2
  Slider Gain : simulink/Math Operations/Slider Gain  SystemSampleTime=-1  low=0  gain=1  high=2
  a : Constant
  a-z : Sum  Inputs=+-  OutScaling=2^-10
  X_w : Outport
  wires:
  X_in/1 -> Product/2
  Product/1 -> X_w/1
  X_Z/1 -> Select z/1
  Select z/1 -> a-z/2
  a-z/1 -> Slider Gain/1
  Constant/1 -> Mux/1, Mux/3, Multiport Switch/2
  a/1 -> a-z/1
  Slider Gain/1 -> Multiport Switch/3
  X_W ON/OFF/1 -> Multiport Switch/1
  Multiport Switch/1 -> Mux/4, Mux/2
  Mux/1 -> Product/1

== system q_3d_crane_cal/Setpoints for  Calibration/Calibration Setpoint: Payload/Setpoint Calibration: Payload ==
  ls payload : Inport
  Go to Home : Constant  Value=sp_home_payload
  Go to Ret : Subsystem
  Latch Payload limit : Subsystem
  Multiport Switch : MultiPortSwitch  Inputs=2  zeroidx=on
  Unit Delay : UnitDelay  SampleTime=qc_get_step_size
  reset : Outport  InitialOutput=0
  xd : Outport  Port=2  InitialOutput=0
  wires:
  Latch Payload limit/1(Latch IN) -> Multiport Switch/1, Unit Delay/1
  ls payload/1 -> Latch Payload limit/1(IN)
  Multiport Switch/1 -> xd/1
  Go to Ret/1(xd (m)) -> Multiport Switch/2
  Go to Home/1 -> Multiport Switch/3
  Unit Delay/1 -> reset/1

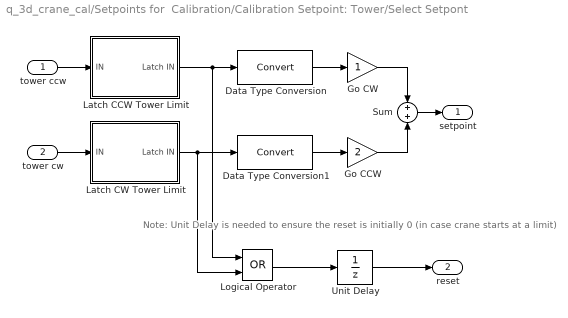
== system q_3d_crane_cal/Setpoints for  Calibration/Calibration Setpoint: Tower/Select Setpont ==
  note: Note: Unit Delay is needed
      | to ensure the reset is initially 0
      | (in case crane starts at a limit)
  tower ccw : Inport
  tower cw : Inport  Port=2
  Data Type Conversion : DataTypeConversion
  Data Type Conversion1 : DataTypeConversion
  Go CCW : Gain  Gain=2
  Go CW : Gain
  Latch CCW Tower Limit : Subsystem
  Latch CW Tower Limit : Subsystem
  Logical Operator : Logic  Operator=OR  AllPortsSameDT=off  OutDataTypeMode=Boolean
  Sum : Sum
  Unit Delay : UnitDelay  SampleTime=qc_get_step_size
  setpoint : Outport
  reset : Outport  Port=2  InitialOutput=0
  wires:
  Latch CCW Tower Limit/1(Latch IN) -> Data Type Conversion/1, Logical Operator/1
  Logical Operator/1 -> Unit Delay/1
  Latch CW Tower Limit/1(Latch IN) -> Data Type Conversion1/1, Logical Operator/2
  Go CCW/1 -> Sum/2
  Data Type Conversion1/1 -> Go CCW/1
  Data Type Conversion/1 -> Go CW/1
  Unit Delay/1 -> reset/1
  tower cw/1 -> Latch CW Tower Limit/1(IN)
  tower ccw/1 -> Latch CCW Tower Limit/1(IN)
  Go CW/1 -> Sum/1
  Sum/1 -> setpoint/1

== system q_3d_crane_cal/Setpoints for  Calibration/Calibration Setpoint: Tower/Start rotating CCW ==
  Amplitude  (deg/s) : Gain  Gain=20.0
  Constant : Constant
  Discrete-Time Integrator : DiscreteIntegrator  SampleTime=qc_get_step_size  ICPrevOutput=DiscIntNeverNeededParam  ICPrevScaledInput=DiscIntNeverNeededParam
  xd (deg) : Outport
  wires:
  Constant/1 -> Discrete-Time Integrator/1
  Discrete-Time Integrator/1 -> Amplitude  (deg/s)/1
  Amplitude  (deg/s)/1 -> xd (deg)/1

== system q_3d_crane_cal/Setpoints for  Calibration/Calibration Setpoint: Trolley/Setpoint Calibration: Trolley ==
  ret : Inport
  Go to Home : Constant  Value=sp_home_trolley
  Go to Ret : Subsystem
  Latch RET limit : Subsystem
  Multiport Switch : MultiPortSwitch  Inputs=2  zeroidx=on
  reset : Outport  InitialOutput=0
  xd : Outport  Port=2  InitialOutput=0
  wires:
  Go to Ret/1(xd (m)) -> Multiport Switch/2
  Go to Home/1 -> Multiport Switch/3
  Multiport Switch/1 -> xd/1
  ret/1 -> Latch RET limit/1(IN)
  Latch RET limit/1(Latch IN) -> reset/1, Multiport Switch/1

== system q_3d_crane_cal/Setpoints for  Calibration/Calibration Setpoint: Payload/Setpoint Calibration: Payload/Go to Ret ==
  Amplitude  (m/s) : Gain  Gain=50e-3
  Discrete-Time Integrator : DiscreteIntegrator  SampleTime=qc_get_step_size  ICPrevOutput=DiscIntNeverNeededParam  ICPrevScaledInput=DiscIntNeverNeededParam
  Go to Ret : Constant
  xd (m) : Outport
  wires:
  Amplitude  (m/s)/1 -> xd (m)/1
  Go to Ret/1 -> Discrete-Time Integrator/1
  Discrete-Time Integrator/1 -> Amplitude  (m/s)/1

== system q_3d_crane_cal/Setpoints for  Calibration/Calibration Setpoint: Payload/Setpoint Calibration: Payload/Latch Payload limit ==
  IN : Inport
  Logical Operator : Logic  Operator=OR  AllPortsSameDT=off
  Memory : Memory  Orientation=left  InheritSampleTime=on
  Latch IN : Outport  InitialOutput=0
  wires:
  IN/1 -> Logical Operator/1
  Memory/1 -> Logical Operator/2
  Logical Operator/1 -> Latch IN/1, Memory/1

== system q_3d_crane_cal/Setpoints for  Calibration/Calibration Setpoint: Tower/Select Setpont/Latch CCW Tower Limit ==
  IN : Inport
  Logical Operator : Logic  Operator=OR  AllPortsSameDT=off
  Memory : Memory  Orientation=left  InheritSampleTime=on
  Latch IN : Outport  InitialOutput=0
  wires:
  Logical Operator/1 -> Memory/1, Latch IN/1
  Memory/1 -> Logical Operator/2
  IN/1 -> Logical Operator/1

== system q_3d_crane_cal/Setpoints for  Calibration/Calibration Setpoint: Tower/Select Setpont/Latch CW Tower Limit ==
  IN : Inport
  Logical Operator : Logic  Operator=OR  AllPortsSameDT=off  OutDataTypeMode=Boolean
  Memory : Memory  Orientation=left  InheritSampleTime=on
  Latch IN : Outport  InitialOutput=0
  wires:
  IN/1 -> Logical Operator/1
  Memory/1 -> Logical Operator/2
  Logical Operator/1 -> Latch IN/1, Memory/1

== system q_3d_crane_cal/Setpoints for  Calibration/Calibration Setpoint: Trolley/Setpoint Calibration: Trolley/Go to Ret ==
  Amplitude  (m/s) : Gain  Gain=50e-3
  Discrete-Time Integrator : DiscreteIntegrator  SampleTime=qc_get_step_size  ICPrevOutput=DiscIntNeverNeededParam  ICPrevScaledInput=DiscIntNeverNeededParam
  Go to Ret : Constant  Value=-1
  xd (m) : Outport
  wires:
  Discrete-Time Integrator/1 -> Amplitude  (m/s)/1
  Go to Ret/1 -> Discrete-Time Integrator/1
  Amplitude  (m/s)/1 -> xd (m)/1

== system q_3d_crane_cal/Setpoints for  Calibration/Calibration Setpoint: Trolley/Setpoint Calibration: Trolley/Latch RET limit ==
  IN : Inport
  Logical Operator : Logic  Operator=OR  AllPortsSameDT=off
  Memory : Memory  Orientation=left  InheritSampleTime=on
  Latch IN : Outport  InitialOutput=0
  wires:
  Logical Operator/1 -> Memory/1, Latch IN/1
  Memory/1 -> Logical Operator/2
  IN/1 -> Logical Operator/1
